simulink library "YMDHMS_2_dec_year"  (R2016b)
settings: Solver=VariableStepAuto  StartTime=0.0  StopTime=10.0  RelTol=1e-3
settings Model: Creator=taylorreynolds  LastModifiedBy=taylorreynolds

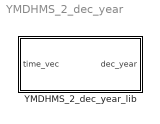
== system YMDHMS_2_dec_year ==
  YMDHMS_2_dec_year_lib : Subsystem

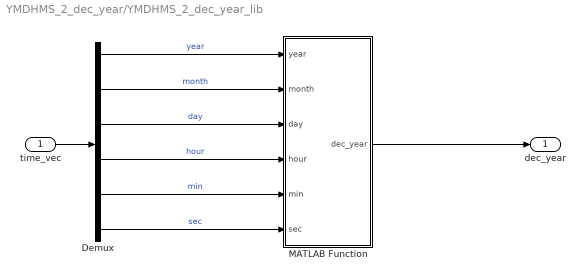
== system YMDHMS_2_dec_year/YMDHMS_2_dec_year_lib ==
  time_vec : Inport
  Demux : Demux  Outputs=6
  MATLAB Function : MATLAB Function  TreatAsAtomicUnit=on
  dec_year : Outport
  wires:
  time_vec/1 -> Demux/1
  Demux/1 -> MATLAB Function/1(year)  "year"
  Demux/2 -> MATLAB Function/2(month)  "month"
  Demux/3 -> MATLAB Function/3(day)  "day"
  Demux/4 -> MATLAB Function/4(hour)  "hour"
  Demux/5 -> MATLAB Function/5(min)  "min"
  Demux/6 -> MATLAB Function/6(sec)  "sec"
  MATLAB Function/1(dec_year) -> dec_year/1

== matlab function YMDHMS_2_dec_year/YMDHMS_2_dec_year_lib/MATLAB Function ==
  data: year input; dec_year output; month input; day input; hour input; min input; sec input
function dec_year = fcn(year,month,day,hour,min,sec)

% UW HuskySat 1, ADCS Subsystem
%   T. Reynolds, Updated: 10.28.17

% Converts a time vector into a decimal year number. See Vallado pp 200-201
% for reference algorithms. Uses 6 inputs to avoid 1 based indexing.

% find day of year - valid until 2100
Lmonth = [31, 28, 31, 30, 31, 30, 31, 31, 30, 31, 30, 31];
days_in_year    = 365.25;

if mod(year,4) == 0
    Lmonth(2) = 29;
    days_in_year    = 366;
end

day_of_year = 0;
for i = 1:month-1
    day_of_year = day_of_year + Lmonth(i);
end

% Add number of days into the month
day_of_year = day_of_year + day;

% Add HMS info to the day of year
day_of_year    = day_of_year + hour/24 + min/1440 + sec/86400;

% Find the year fraction represented by day_of_year
day_frac    = day_of_year/days_in_year;

% Sum to get total decimal year
dec_year = year + day_frac;

end
